simulink model "ThreePhaseInverter120degrees"  (R2018a)
settings: Solver=VariableStepAuto  StartTime=0.0  StopTime=10.0  RelTol=1e-3
libraries: powerlib x15
settings Model: Creator=Bhaskar  LastModifiedBy=Bhaskar

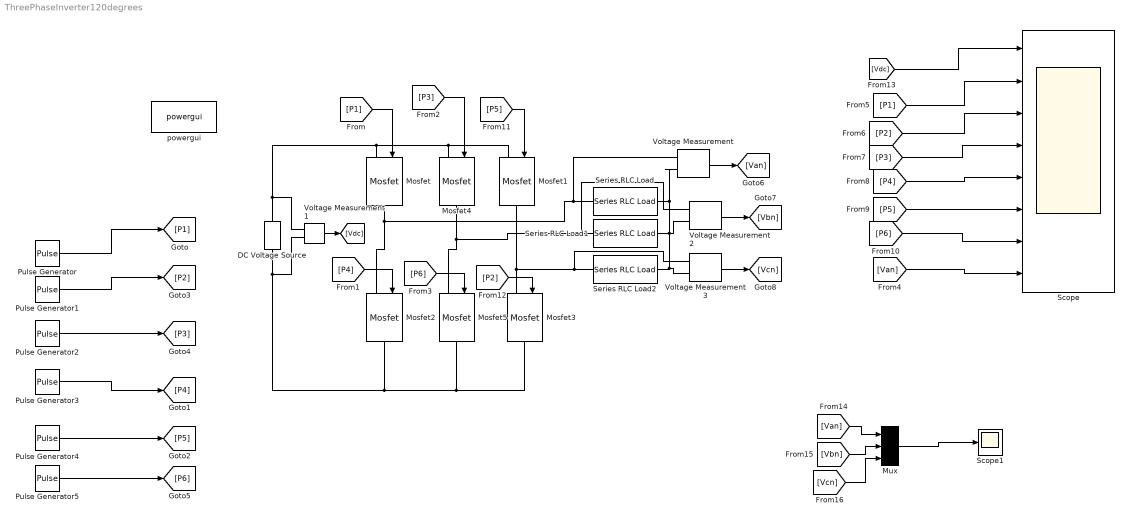
== system ThreePhaseInverter120degrees ==
  DC Voltage Source : powerlib/Electrical Sources/DC Voltage Source  Amplitude=100  Measurements=None
  Mosfet{,1..5} (6 alike) : powerlib/Power Electronics/Mosfet  Ron=0.1  Lon=0  Rd=0.01  Vfd=0  IC=0  Rs=1e5  Cs=inf  Measurements=off
  Mux : Mux  Inputs=3
  Pulse Generator : DiscretePulseGenerator  PulseType=Time based  Period=1/50  PulseWidth=(120/360)*100
  Pulse Generator1 : DiscretePulseGenerator  PulseType=Time based  Period=1/50  PulseWidth=(120/360)*100  PhaseDelay=60*(1/50/360)
  Pulse Generator2 : DiscretePulseGenerator  PulseType=Time based  Period=1/50  PulseWidth=(120/360)*100  PhaseDelay=120*(1/50/360)
  Pulse Generator3 : DiscretePulseGenerator  PulseType=Time based  Period=1/50  PulseWidth=(120/360)*100  PhaseDelay=180*(1/50/360)
  Pulse Generator4 : DiscretePulseGenerator  PulseType=Time based  Period=1/50  PulseWidth=(120/360)*100  PhaseDelay=240*(1/50/360)
  Pulse Generator5 : DiscretePulseGenerator  PulseType=Time based  Period=1/50  PulseWidth=(120/360)*100  PhaseDelay=300*(1/50/360)
  Scope : Scope  NumInputPorts=8
  Scope1 : Scope
  Series RLC Load : powerlib/Elements/Series RLC Load  LConnTagsString=a  RConnTagsString=__new0  NominalVoltage=230  NominalFrequency=50  ActivePower=1000  InductivePower=0  CapacitivePower=0  Setx0=off  InitialVoltage=0  SetiL0=off  InitialCurrent=0  Measurements=None  LoadType=constant Z
  Series RLC Load1 : powerlib/Elements/Series RLC Load  LConnTagsString=a  RConnTagsString=__new0  NominalVoltage=230  NominalFrequency=50  ActivePower=1000  InductivePower=0  CapacitivePower=0  Setx0=off  InitialVoltage=0  SetiL0=off  InitialCurrent=0  Measurements=None  LoadType=constant Z
  Series RLC Load2 : powerlib/Elements/Series RLC Load  LConnTagsString=a  RConnTagsString=__new0  NominalVoltage=230  NominalFrequency=50  ActivePower=1000  InductivePower=0  CapacitivePower=0  Setx0=off  InitialVoltage=0  SetiL0=off  InitialCurrent=0  Measurements=None  LoadType=constant Z
  Voltage Measurement{,1..3} (4 alike) : powerlib/Measurements/Voltage Measurement  PhasorSimulation=off  OutputType=Complex  PSBequivalent=0
  powergui : powerlib/powergui  Priority=1  SimulationMode=Discrete  SampleTime=50e-6  frequency=60  Iterations=50  frequencyindice=0  Pbase=100e6  ErrMax=1e-4  UnitsV=kV  UnitsW=MW  buscounter=0  FunctionMessages=off  echomessages=off  EnableUseOfTLC=off  CurrentSourceSwitches=off  DisableSnubberDevices=off  DisableRonSwitches=off  DisableVfSwitches=off  DisplayEquations=off  SolverType=Tustin/Backward Euler (TBE)  Interpol=off  ExternalGateDelay=off  methode=off  Ts=100  x0status=blocks  SPID=off  SwTol=0  HookPort=off  RestoreLinks=warning  ResistiveCurrentMeasurement=off  Frange=[0:2:500]  Ylog=off  Xlog=on  ShowGrid=off  save=off  variable=ZData  structure=0  ZoomFFT=off  StartTime=0.0  cycles=1  DisplayStyle=1  fundamental=60  FreqAxis=off  MaxFrequency=1000  frequencyindicesteady=1  RmsSteady=1  display=off
  wires:
  Voltage Measurement1/1 -> [Vdc]
  [P1] -> Scope/2
  [P4] -> Scope/5
  [Vdc] -> Scope/1
  [P6] -> Scope/7
  [P4] -> Mosfet2/1
  [P2] -> Mosfet3/1
  [Vcn] -> Mux/3
  Mux/1 -> Scope1/1
  [Vbn] -> Mux/2
  Voltage Measurement3/1 -> [Vcn]
  [P1] -> Mosfet/1
  [P3] -> Scope/4
  [P2] -> Scope/3
  Voltage Measurement/1 -> [Van]
  [P5] -> Scope/6
  [P5] -> Mosfet1/1
  [P3] -> Mosfet4/1
  [Van] -> Mux/1
  Voltage Measurement2/1 -> [Vbn]
  [Van] -> Scope/8
  [P6] -> Mosfet5/1
  Pulse Generator/1 -> [P1]
  Pulse Generator1/1 -> [P2]
  Pulse Generator2/1 -> [P3]
  Pulse Generator3/1 -> [P4]
  Pulse Generator4/1 -> [P5]
  Pulse Generator5/1 -> [P6]
  connections:
  Mosfet2/RConn1 -- Mosfet5/RConn1 -- Mosfet3/RConn1 -- Voltage Measurement1/LConn2 -- DC Voltage Source/LConn1
  Mosfet3/LConn1 -- Voltage Measurement3/LConn1 -- Series RLC Load2/RConn1 -- Mosfet1/RConn1
  DC Voltage Source/RConn1 -- Voltage Measurement1/LConn1 -- Mosfet4/LConn1 -- Mosfet1/LConn1 -- Mosfet/LConn1
  Series RLC Load1/LConn1 -- Voltage Measurement2/LConn2 -- Voltage Measurement/LConn2 -- Series RLC Load/LConn1 -- Voltage Measurement3/LConn2 -- Series RLC Load2/LConn1
  Series RLC Load1/RConn1 -- Voltage Measurement2/LConn1 -- Mosfet5/LConn1 -- Mosfet4/RConn1
  Mosfet2/LConn1 -- Voltage Measurement/LConn1 -- Series RLC Load/RConn1 -- Mosfet/RConn1
